simulink model "trimtest_with_vector_outport"  (Simulink 2.20)
settings: Solver=ode45  StartTime=0.0  StopTime=20  RelTol=1e-3  AbsTol=1e-6
StartFcn:
  | rand; global x_tr
undefined symbols (not defined in the file or in its folder): i
libraries: simulink x3
CloseFcn:
  | ;slview('closediagram',bdroot);
settings Model: LoadExternalInput=on  ExternalInput=[0 0 0 0 0 0 0 0 0]  LoadInitialState=on  InitialState=[0;0;0;0;0;0;0;0;0;0;0;0;0;0]  ConsistencyChecking=off  RTWPlaceOutputsASAP=off  RTWTemplateMakefile=grt_vc.tmf

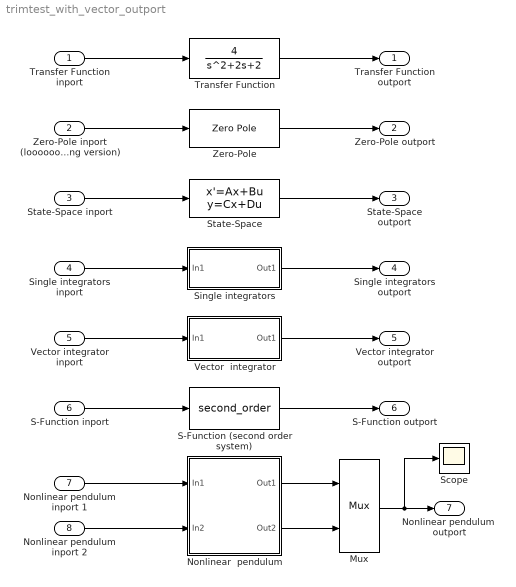
== system trimtest_with_vector_outport ==
  Transfer Function inport : Inport  Port=1  PortWidth=-1  SampleTime=-1
  Zero-Pole inport (looooooooooooooooooooooooooong version) : Inport  Port=2  PortWidth=-1  SampleTime=-1
  State-Space inport : Inport  Port=3  PortWidth=-1  SampleTime=-1
  Single integrators inport : Inport  Port=4  PortWidth=-1  SampleTime=-1
  Vector integrator inport : Inport  Port=5  PortWidth=-1  SampleTime=-1
  S-Function inport : Inport  Port=6  PortWidth=-1  SampleTime=-1
  Nonlinear pendulum inport 1 : Inport  Port=7  PortWidth=-1  SampleTime=-1
  Nonlinear pendulum inport 2 : Inport  Port=8  PortWidth=-1  SampleTime=-1
  Mux : Mux  Inputs=2
  Nonlinear  pendulum : Subsystem
  S-Function (second order system) : S-Function  FunctionName=second_order  PortCounts=[]  SFunctionModules=''
  Scope : Scope
      settings: TickLabels=on  TimeRange=auto  YMin=0  YMax=180  SaveToWorkspace=off  SaveName=ScopeData
  Single integrators : Subsystem
  State-Space : StateSpace  A=[0, 1; -2, -2]  B=[0; 4]  C=[1, 0]  D=0  X0=0
  Transfer Function : TransferFcn  Numerator=4  Denominator=[1, 2, 2]
  Vector  integrator : Subsystem
  Zero-Pole : ZeroPole  Zeros=[]  Poles=[-1+i; -1-i]  Gain=4
  Transfer Function outport : Outport  Port=1
  Zero-Pole outport : Outport  Port=2
  State-Space outport : Outport  Port=3
  Single integrators outport : Outport  Port=4
  Vector integrator outport : Outport  Port=5
  S-Function outport : Outport  Port=6
  Nonlinear pendulum  outport : Outport  Port=7
  wires:
  Vector integrator inport/1 -> Vector  integrator/1(In1)
  S-Function inport/1 -> S-Function (second order system)/1
  Single integrators inport/1 -> Single integrators/1(In1)
  Transfer Function inport/1 -> Transfer Function/1
  Zero-Pole inport (looooooooooooooooooooooooooong version)/1 -> Zero-Pole/1
  State-Space inport/1 -> State-Space/1
  Nonlinear pendulum inport 1/1 -> Nonlinear  pendulum/1(In1)
  Nonlinear pendulum inport 2/1 -> Nonlinear  pendulum/2(In2)
  Vector  integrator/1(Out1) -> Vector integrator outport/1
  Single integrators/1(Out1) -> Single integrators outport/1
  S-Function (second order system)/1 -> S-Function outport/1
  State-Space/1 -> State-Space outport/1
  Transfer Function/1 -> Transfer Function outport/1
  Zero-Pole/1 -> Zero-Pole outport/1
  Nonlinear  pendulum/1(Out1) -> Mux/1
  Nonlinear  pendulum/2(Out2) -> Mux/2
  Mux/1 -> Nonlinear pendulum  outport/1, Scope/1

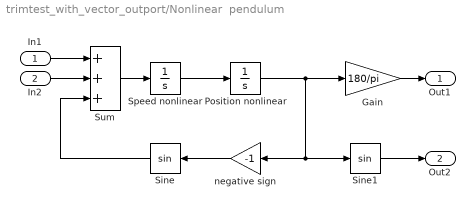
== system trimtest_with_vector_outport/Nonlinear  pendulum ==
  In1 : Inport  Port=1  PortWidth=-1  SampleTime=-1
  In2 : Inport  Port=2  PortWidth=-1  SampleTime=-1
  Gain : Gain  Gain=180/pi
  Position nonlinear : Integrator  ExternalReset=none  InitialConditionSource=internal  InitialCondition=0  LimitOutput=off  UpperSaturationLimit=inf  LowerSaturationLimit=-inf  ShowSaturationPort=off  ShowStatePort=off  AbsoluteTolerance=auto
  Sine : Trigonometry  Orientation=left  Operator=sin
  Sine1 : Trigonometry  Operator=sin
  Speed nonlinear : Integrator  ExternalReset=none  InitialConditionSource=internal  InitialCondition=0  LimitOutput=off  UpperSaturationLimit=inf  LowerSaturationLimit=-inf  ShowSaturationPort=off  ShowStatePort=off  AbsoluteTolerance=auto
  Sum : Sum  Inputs=3
  negative sign : Gain  Orientation=left  Gain=-1
  Out1 : Outport  Port=1  InitialOutput=0
  Out2 : Outport  Port=2  InitialOutput=0
  wires:
  negative sign/1 -> Sine/1
  Speed nonlinear/1 -> Position nonlinear/1
  Position nonlinear/1 -> Gain/1, negative sign/1, Sine1/1
  Gain/1 -> Out1/1
  Sine1/1 -> Out2/1
  Sum/1 -> Speed nonlinear/1
  Sine/1 -> Sum/3
  In1/1 -> Sum/1
  In2/1 -> Sum/2

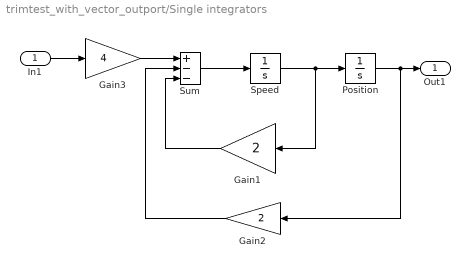
== system trimtest_with_vector_outport/Single integrators ==
  In1 : Inport  Port=1  PortWidth=-1  SampleTime=-1
  Gain1 : Gain  Orientation=left  Gain=2
  Gain2 : Gain  Orientation=left  Gain=2
  Gain3 : Gain  Gain=4
  Position : Integrator  ExternalReset=none  InitialConditionSource=internal  InitialCondition=0  LimitOutput=off  UpperSaturationLimit=inf  LowerSaturationLimit=-inf  ShowSaturationPort=off  ShowStatePort=off  AbsoluteTolerance=auto
  Speed : Integrator  ExternalReset=none  InitialConditionSource=internal  InitialCondition=0  LimitOutput=off  UpperSaturationLimit=inf  LowerSaturationLimit=-inf  ShowSaturationPort=off  ShowStatePort=off  AbsoluteTolerance=auto
  Sum : Sum  Inputs=+--
  Out1 : Outport  Port=1  InitialOutput=0
  wires:
  In1/1 -> Gain3/1
  Sum/1 -> Speed/1
  Gain1/1 -> Sum/3
  Speed/1 -> Position/1, Gain1/1
  Gain2/1 -> Sum/2
  Position/1 -> Gain2/1, Out1/1
  Gain3/1 -> Sum/1

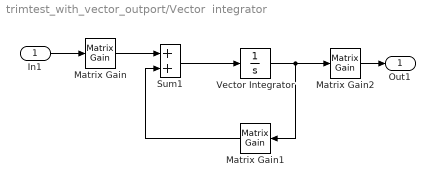
== system trimtest_with_vector_outport/Vector  integrator ==
  In1 : Inport  Port=1  PortWidth=-1  SampleTime=-1
  Matrix Gain : simulink/Linear/Matrix Gain  K=[0; 4]
  Matrix Gain1 : simulink/Linear/Matrix Gain  Orientation=left  K=[0, 1; -2, -2]
  Matrix Gain2 : simulink/Linear/Matrix Gain  K=[1, 0]
  Sum1 : Sum  Inputs=++
  Vector Integrator : Integrator  ExternalReset=none  InitialConditionSource=internal  InitialCondition=[0 0]  LimitOutput=off  UpperSaturationLimit=inf  LowerSaturationLimit=-inf  ShowSaturationPort=off  ShowStatePort=off  AbsoluteTolerance=auto
  Out1 : Outport  Port=1  InitialOutput=0
  wires:
  In1/1 -> Matrix Gain/1
  Sum1/1 -> Vector Integrator/1
  Matrix Gain/1 -> Sum1/1
  Vector Integrator/1 -> Matrix Gain2/1, Matrix Gain1/1
  Matrix Gain1/1 -> Sum1/2
  Matrix Gain2/1 -> Out1/1
